simulink model "BOOST_PFC"  (R2022a)
settings: Solver=VariableStepAuto  StartTime=0.0  StopTime=1.5  FixedStep=1e-6  RelTol=1e-3
libraries: spsVoltageMeasurementLib x7, spsCurrentMeasurementLib x5, spsDiodeLib x5, spsSeriesRLCBranchLib x3, spsACVoltageSourceLib x1, spsMosfetLib x1, slpidlib x1, spsPWMGeneratorDCDCLib x1, spsRMSLib x1, simulink_extras x1, spspowerguiLib x1
settings Model: Creator=ASUS  LastModifiedBy=Swastik Sharma
settings DataIOCC: SaveFormat=StructureWithTime  ReturnWorkspaceOutputs=off
settings DebuggingCC: SignalInfNanChecking=error  UnconnectedInputMsg=warning  UnconnectedOutputMsg=warning  UnconnectedLineMsg=warning
settings RTWCC: DLArmComputeVersion=19.05

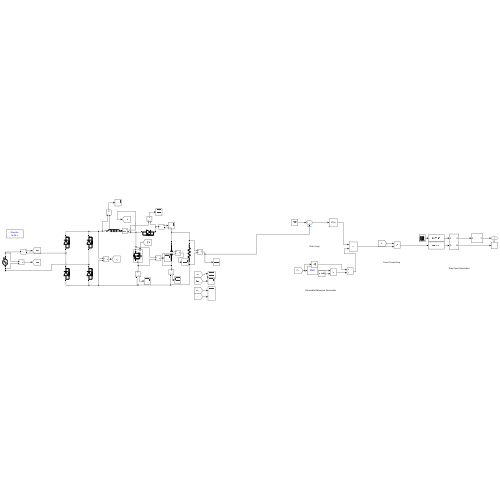
[thumbnail: Simulink's stored preview of the top-level diagram]
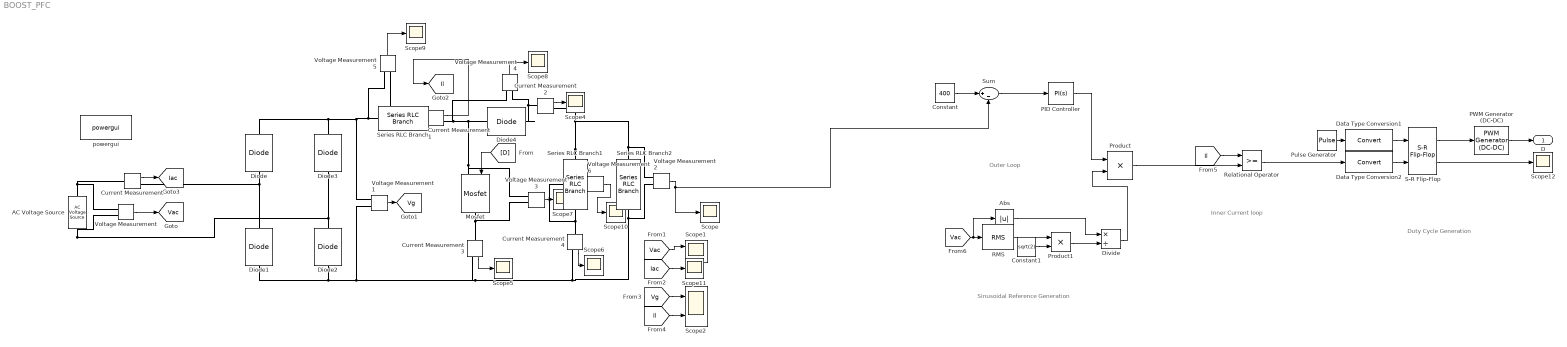
== system BOOST_PFC ==
  note: Outer Loop
  note: Sinusoidal Reference Generation
  note: Duty Cycle Generation
  note: Inner Current loop
  AC Voltage Source : spsACVoltageSourceLib/AC Voltage Source  Amplitude=325  Phase=0  Frequency=50  SampleTime=0  Measurements=None  BusType=swing  Pref=10e3  Qref=0  Qmin=-inf  Qmax=+inf
  Abs : Abs  SaturateOnIntegerOverflow=off
  Constant : Constant  Value=400
  Constant1 : Constant  Value=sqrt(2)
  Current Measurement{,1..4} (5 alike) : spsCurrentMeasurementLib/Current Measurement  PhasorSimulation=off  OutputType=Complex  PSBequivalent=0
  Data Type Conversion1 : DataTypeConversion  SaturateOnIntegerOverflow=off  RndMeth=Floor
  Data Type Conversion2 : DataTypeConversion  SaturateOnIntegerOverflow=off  RndMeth=Floor
  Diode{,1..4} (5 alike) : spsDiodeLib/Diode  Ron=0.001  Lon=0  Vf=0.7  IC=0  UseSnubber=0  Rs=500  Cs=250e-9  Measurements=off
  Divide : Product  Inputs=*/
  Mosfet : spsMosfetLib/Mosfet  Ron=0.1  Lon=0  Rd=0.01  Vfd=0  IC=0  Rs=1e5  Cs=inf  Measurements=off
  PID Controller : slpidlib/PID Controller  Controller=PI  Form=Parallel  TimeDomain=Continuous-time  UseExternalTs=off  SampleTime=-1  IntegratorMethod=Forward Euler  FilterMethod=Forward Euler  ControllerParametersSource=internal  P=0.14  I=3.632  UseKiTs=off  D=-1.721584044714349e-04  N=100  UseFilter=on  TunerSelectOption=Transfer Function Based (PID Tuner App)  InitialConditionSource=internal  InitialConditionForIntegrator=0  InitialConditionForFilter=0  DifferentiatorICPrevScaledInput=0  ExternalReset=none  TrackingMode=off  Kt=1  LimitOutput=off  SatLimitsSource=internal  UpperSaturationLimit=25  LowerSaturationLimit=0  LinearizeAsGain=on  AntiWindupMode=none  Kb=1  POutMin=[]  POutMax=[]  IOutMin=[]  IOutMax=[]  DOutMin=[]  DOutMax=[]  NOutMin=[]  NOutMax=[]  SumOutMin=[]  SumOutMax=[]  SaturationOutMin=[]  SaturationOutMax=[]  PParamMin=[]  PParamMax=[]  IParamMin=[]  IParamMax=[]  DParamMin=[]  DParamMax=[]  NParamMin=[]  NParamMax=[]  KbParamMin=[]  KbParamMax=[]  KtParamMin=[]  KtParamMax=[]  KbOutMin=[]  KbOutMax=[]  KtOutMin=[]  KtOutMax=[]  IntegratorOutMin=[]  IntegratorOutMax=[]  FilterOutMin=[]  FilterOutMax=[]  SumI1OutMin=[]  SumI1OutMax=[]  SumI2OutMin=[]  SumI2OutMax=[]  SumI3OutMin=[]  SumI3OutMax=[]  SumI4OutMin=[]  SumI4OutMax=[]  SumDOutMin=[]  SumDOutMax=[]  DifferentiatorOutMin=[]  DifferentiatorOutMax=[]  FilterDiffOutCoefMin=[]  FilterDiffOutCoefMax=[]  ReciprocalOutMin=[]  ReciprocalOutMax=[]  SumDenOutMin=[]  SumDenOutMax=[]  SumNumOutMin=[]  SumNumOutMax=[]  DivideOutMin=[]  DivideOutMax=[]  UdiffTsProdOutMin=[]  UdiffTsProdOutMax=[]  NTsProdOutMin=[]  NTsProdOutMax=[]  UintegralTsProdOutMin=[]  UintegralTsProdOutMax=[]  UngainTsProdOutMin=[]  UngainTsProdOutMax=[]  IntegratorContinuousStateAttributes=''  IntegratorStateMustResolveToSignalObject=off  IntegratorRTWStateStorageClass=Auto  FilterContinuousStateAttributes=''  FilterStateMustResolveToSignalObject=off  FilterRTWStateStorageClass=Auto  ParallelPVariant=InternalParameters  IdealPVariant=Disabled  IVariant=InternalParameters  DVariant=Disabled  IntegratorVariant=Continuous  SatVariant=Disabled  AWVariant=Passthrough  PCopyVariant=Disabled  TRVariant=Disabled  FdbkBlocksVariant=Forward  IdealPFdbkVariant=Disabled  SatFdbkVariant=Disabled  DerivativeFilterVariant=Disabled  NVariant=Disabled  NCopyVariant=Disabled_SignalSpec  FilterICVariant=Disabled  IntegratorICVariant=InternalICs  ExternalResetVariant=Disabled  TRSumVariant=Passthrough  SumFdbkVariant=Disabled  SumVariant=Sum_PI  TsampFilterVariant=InternalTs  TsampNgainVariant=Passthrough  TsampIntegralVariant=Passthrough  ExternalSaturationOutDataTypeStr=Inherit: Same as second input  aMode=0
  PWM Generator (DC-DC) : spsPWMGeneratorDCDCLib/PWM Generator (DC-DC)  Fsw=50000  Ts=1e-6
  Product : Product
  Product1 : Product
  Pulse Generator : DiscretePulseGenerator  PulseType=Time based  Period=1.538e-5  PulseWidth=10
  RMS : spsRMSLib/RMS  TrueRMS=on  Freq=50  RMSInit=230  Ts=0
  Relational Operator : RelationalOperator  OutDataTypeStr=boolean  RndMeth=Simplest  InputSameDT=off
  S-R Flip-Flop : simulink_extras/Flip Flops/S-R Flip-Flop  initial_condition=0
  Scope{,4..12} (10 alike) : Scope
  Scope1 : Scope  NumInputPorts=2
  Scope2 : Scope  NumInputPorts=2
  Series RLC Branch : spsSeriesRLCBranchLib/Series RLC Branch  LConnTagsString=__new0  RConnTagsString=__new0  BranchType=L  Resistance=1  Inductance=3.2e-3  SetiL0=off  InitialCurrent=0  Capacitance=1e-6  Setx0=off  InitialVoltage=0  Measurements=None
  Series RLC Branch1 : spsSeriesRLCBranchLib/Series RLC Branch  LConnTagsString=__new0  RConnTagsString=__new0  BranchType=C  Resistance=1  Inductance=1e-3  SetiL0=off  InitialCurrent=0  Capacitance=10e-3  Setx0=off  InitialVoltage=0  Measurements=None
  Series RLC Branch2 : spsSeriesRLCBranchLib/Series RLC Branch  LConnTagsString=__new0  RConnTagsString=__new0  BranchType=R  Resistance=400/3  Inductance=1e-3  SetiL0=off  InitialCurrent=0  Capacitance=1e-6  Setx0=off  InitialVoltage=0  Measurements=None
  Sum : Sum  Inputs=|+-
  Voltage Measurement{,1..6} (7 alike) : spsVoltageMeasurementLib/Voltage Measurement  PhasorSimulation=off  OutputType=Complex  PSBequivalent=0
  powergui : spspowerguiLib/powergui  Priority=1  SimulationMode=Discrete  SampleTime=1e-6  frequency=60  Iterations=50  frequencyindice=50  Pbase=100e6  ErrMax=1e-4  UnitsV=kV  UnitsW=MW  buscounter=0  FunctionMessages=off  echomessages=off  EnableUseOfTLC=off  CurrentSourceSwitches=off  DisableSnubberDevices=off  DisableRonSwitches=off  DisableVfSwitches=off  DisplayEquations=off  AutomaticDiscreteSolvers=off  SolverType=Tustin/Backward Euler (TBE)  Interpol=off  ExternalGateDelay=off  methode=off  Ts=100  x0status=blocks  SPID=on  SwTol=0  HookPort=off  NonlinearTolerance=1e-4  nMaxIteration=100  ContinueOnMaxIteration=off  RestoreLinks=warning  ResistiveCurrentMeasurement=off  Frange=[0:2:500]  Ylog=off  Xlog=on  ShowGrid=off  save=off  variable=ZData  structure=0  ZoomFFT=off  StartTime=0.0  cycles=1  DisplayStyle=1  fundamental=60  FreqAxis=off  MaxFrequency=1000  frequencyindicesteady=1  RmsSteady=1  display=off
  D : Outport
  tag scope: Iac=global, Il=global, Vac=global, Vg=global
  wires:
  Voltage Measurement/1 -> [Vac]
  Voltage Measurement1/1 -> [Vg]
  [D] -> Mosfet/1
  Current Measurement1/1 -> [Il]
  Current Measurement/1 -> [Iac]
  Voltage Measurement2/1 -> Sum/2, Scope/1
  [Vac] -> Scope1/1
  [Vg] -> Scope2/1
  [Il] -> Scope2/2
  Current Measurement2/1 -> Scope4/1
  Current Measurement3/1 -> Scope5/1
  Current Measurement4/1 -> Scope6/1
  Voltage Measurement3/1 -> Scope7/1
  Voltage Measurement4/1 -> Scope8/1
  Voltage Measurement5/1 -> Scope9/1
  Voltage Measurement6/1 -> Scope10/1
  [Iac] -> Scope11/1
  Product/1 -> Relational Operator/2
  PWM Generator (DC-DC)/1 -> D/1
  Constant1/1 -> Product1/2
  Divide/1 -> Product/2
  S-R Flip-Flop/1 -> PWM Generator (DC-DC)/1
  Data Type Conversion2/1 -> S-R Flip-Flop/2
  Relational Operator/1 -> Data Type Conversion2/1
  Product1/1 -> Divide/2
  RMS/1 -> Product1/1
  Data Type Conversion1/1 -> S-R Flip-Flop/1
  [Vac] -> Abs/1, RMS/1
  Abs/1 -> Divide/1
  [Il] -> Relational Operator/1
  Pulse Generator/1 -> Data Type Conversion1/1
  S-R Flip-Flop/2 -> Scope12/1
  Sum/1 -> PID Controller/1
  PID Controller/1 -> Product/1
  Constant/1 -> Sum/1
  connections:
  Diode/LConn1 -- Current Measurement/RConn1 -- Diode1/RConn1
  Diode3/LConn1 -- Voltage Measurement/LConn2 -- AC Voltage Source/LConn1 -- Diode2/RConn1
  Diode/RConn1 -- Voltage Measurement5/LConn1 -- Series RLC Branch/LConn1 -- Voltage Measurement1/LConn1 -- Diode3/RConn1
  Diode4/LConn1 -- Voltage Measurement4/LConn1 -- Current Measurement1/RConn1 -- Voltage Measurement3/LConn1 -- Mosfet/LConn1
  Voltage Measurement2/LConn1 -- Series RLC Branch2/RConn1 -- Current Measurement2/RConn1 -- Voltage Measurement6/LConn1 -- Series RLC Branch1/LConn1
  AC Voltage Source/RConn1 -- Current Measurement/LConn1 -- Voltage Measurement/LConn1
  Current Measurement1/LConn1 -- Series RLC Branch/RConn1 -- Voltage Measurement5/LConn2
  Series RLC Branch2/LConn1 -- Current Measurement4/RConn1 -- Current Measurement3/RConn1 -- Diode1/LConn1 -- Diode2/LConn1 -- Voltage Measurement1/LConn2 -- Voltage Measurement2/LConn2
  Diode4/RConn1 -- Voltage Measurement4/LConn2 -- Current Measurement2/LConn1
  Current Measurement3/LConn1 -- Voltage Measurement3/LConn2 -- Mosfet/RConn1
  Series RLC Branch1/RConn1 -- Voltage Measurement6/LConn2 -- Current Measurement4/LConn1
